simulink library "CTRL_BASECTRL_SKY"  (R2024b)
settings: Solver=VariableStepAuto  StartTime=0.0  StopTime=10.0  RelTol=1e-3
settings Model: Creator=blatak  LastModifiedBy=blatak

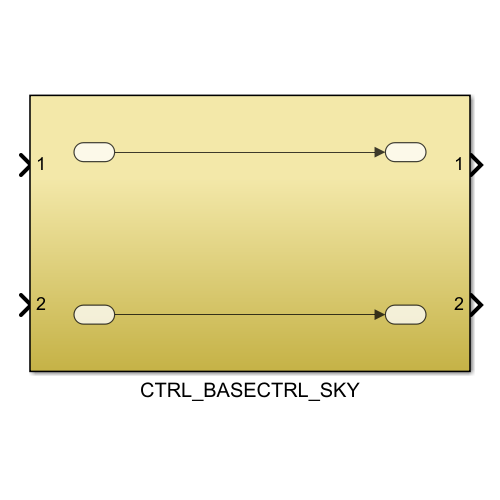
[thumbnail: Simulink's stored preview of the top-level diagram]
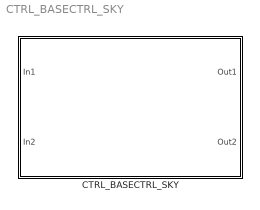
== system CTRL_BASECTRL_SKY ==
  CTRL_BASECTRL_SKY : Subsystem

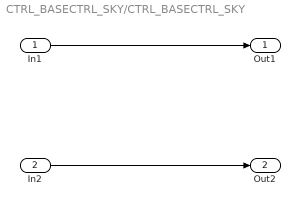
== system CTRL_BASECTRL_SKY/CTRL_BASECTRL_SKY ==
  In1 : Inport
  In2 : Inport  Port=2
  Out1 : Outport
  Out2 : Outport  Port=2
  wires:
  In2/1 -> Out2/1
  In1/1 -> Out1/1
